simulink library "halout"  (R2021b)
settings: Solver=VariableStepAuto  StartTime=0.0  StopTime=10.0  RelTol=1e-3
undefined symbols (not defined in the file): C_TASK_5MS_S, FALSE, KHAL_CAN1TxReq_flg, KHAL_CAN2TxReq_flg, KHAL_CAN3FD3VCU1toNIDECTxReq_flg, KHAL_CAN3FD3VCU1TxReq_flg, KHAL_CAN3FD3VCU2E2E_flg, KHAL_CAN3FD3VCU2toNIDECE2E_flg, KHAL_CAN3FD3VCU2toNIDECTxReq_flg, KHAL_CAN3FD3VCU2TxReq_flg, KHAL_CAN3TxReq_flg, KHAL_CAN4FD4CE1000E2E_flg, KHAL_CAN4FD4CE1000TxReq_flg, KHAL_CAN4TxReq_flg, KHAL_CAN5TxReq_flg, KHAL_CAN7TxReq_flg, ONE_INT, TRUE, ZERO_INT
libraries: FVT_lib x258, simulink x115
(part 3 of 17)

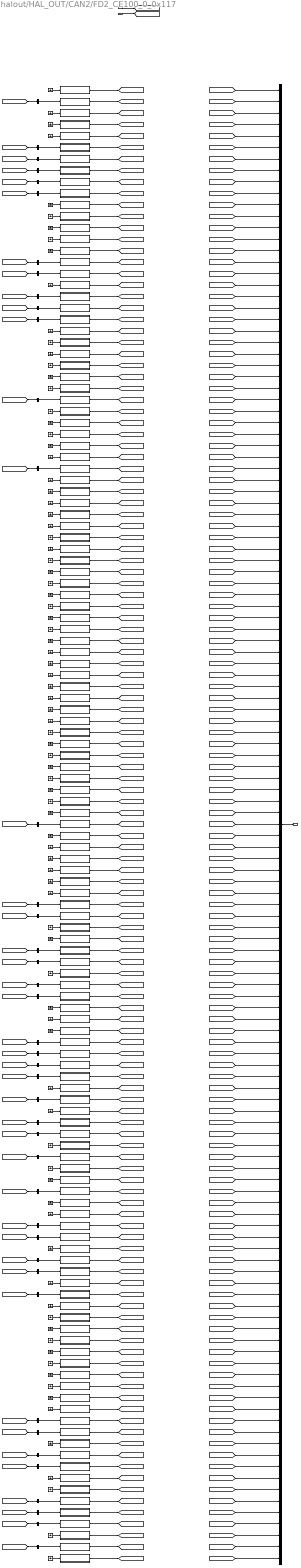
== system halout/HAL_OUT/CAN2/FD2_CE100_0_0x117 ==
  BSCP_outputs : Inport  OutDataTypeStr=Bus: BSCP_outputs
  BOUTP_outputs : Inport  Port=2  OutDataTypeStr=Bus: BOUTP_outputs
  APMDoorControlSta : Subsystem
  ActAPSPosn : Subsystem
  AllDoorSW : Subsystem
  AntitheftSta : Subsystem
  BCMDoorLockSta : Subsystem
  BrakeLamp : Subsystem
  CCCrlSta : Subsystem
  CCMSASpdWar : Subsystem
  CCUACLampSts : Subsystem
  CCUACMaxLampSts : Subsystem
  CCUAutoLampSts : Subsystem
  CCUAutoMidLampSts : Subsystem
  CCUDispalyRequest : Subsystem
  CCUEcoSts : Subsystem
  CCUFrtOnOffLampSts : Subsystem
  CCURrOnOffLampSts : Subsystem
  CCUSyncLampSts : Subsystem
  CoastDwModeStaChk : Subsystem
  CreepSWSta : Subsystem
  DISCButtSta : Subsystem
  DISCSta : Subsystem
  DemoModeStaChk : Subsystem
  Dimmer : Subsystem
  DimmerEN : Subsystem
  DisengagePFail : Subsystem
  DoorLockIND : Subsystem
  DrDoorSW : Subsystem
  DrSeatSta : Subsystem
  DynoModeStaChk : Subsystem
  EDriveSysErrAccPedalErr : Subsystem
  EDriveSysErrMCUErr : Subsystem
  EDriveSysErrShifterErr : Subsystem
  EDriveSysErrVCUErr : Subsystem
  EVDriveMode : Subsystem
  EngActvDmpDisabSta : Subsystem
  EngCoastDwSta : Subsystem
  EngPwrLockSta : Subsystem
  EngagePFail : Subsystem
  FDABSWarning : Subsystem
  FDBatteryChargeWarning : Subsystem
  FDCTHCMCLEVentYSta : Subsystem
  FDCTHCMCLEVentZSta : Subsystem
  FDCTHCMCLVentSta : Subsystem
  FDCTHCMCREVentYSta : Subsystem
  FDCTHCMCREVentZSta : Subsystem
  FDCTHCMCRVentSta : Subsystem
  FDCTHCMDrEVentModeSta : Subsystem
  FDCTHCMDrEVentYSta : Subsystem
  FDCTHCMDrEVentZSta : Subsystem
  FDCTHCMDrVentSta : Subsystem
  FDCTHCMPsEVentModeSta : Subsystem
  FDCTHCMPsEVentYSta : Subsystem
  FDCTHCMPsEVentZSta : Subsystem
  FDCTHCMPsVentSta : Subsystem
  FDCVCUPwrSaveReqCmd : Subsystem
  FDEDriveSystem : Subsystem
  FDEPBError : Subsystem
  FDHVBatteryFault : Subsystem
  FDParkBrakeWarning : Subsystem
  FDPowerlimitation : Subsystem
  FDSteeringWarning : Subsystem
  FDTCSIndicator : Subsystem
  FDTelltaleFail : Subsystem
  FalseNPreventSta : Subsystem
  FeatSetSpdFinalraw32 : Subsystem
  FollowMe : Subsystem
  FrFogLamp : Subsystem
  Ground{,1..86} (87 alike) : Ground
  HBeam : Subsystem
  HVRlyOpFail : Subsystem
  HVSysErrIsolationErr : Subsystem
  HVSysErrPackErr : Subsystem
  HVSysErrRelayErr : Subsystem
  HazardSW : Subsystem
  HoodSW : Subsystem
  LBSD : Subsystem
  LBeam : Subsystem
  LDRL : Subsystem
  LTurnLP : Subsystem
  LVChrgFuncStaChk : Subsystem
  LVSysErrPwrOutpErr : Subsystem
  LimphomeAct : Subsystem
  LockSetting : Subsystem
  MCUActDisFail : Subsystem
  MSACrlSta : Subsystem
  MeterIndSpeedraw32 : Subsystem
  PASStaFSys : Subsystem
  PosLamp : Subsystem
  PsDoorSW : Subsystem
  PwrSta : Subsystem
  PwrStaErr : Subsystem
  PwrStaONTOIVIPopReq : Subsystem
  PwrStaONTOIVIPopT : Subsystem
  RBSD : Subsystem
  RDRL : Subsystem
  RLDoorSW : Subsystem
  RRDoorSW : Subsystem
  RTurnLP : Subsystem
  ReqInternalV2LStatusLamp : Subsystem
  ReqV2LIVIPopup : Subsystem
  ReqV2LSwOn : Subsystem
  ReverseLamp : Subsystem
  RrDefog : Subsystem
  RrFogLamp : Subsystem
  ShiftGearPosn : Subsystem
  SysAllowReadySta : Subsystem
  SysPwrSta : Subsystem
  TailgateSW : Subsystem
  VCUBrkSWSta : Subsystem
  VCUFLDoorSta : Subsystem
  VCUFRDoorSta : Subsystem
  VCUHoodSWSta : Subsystem
  VCUOPDHold : Subsystem
  VCURLDoorSta : Subsystem
  VCURRDoorSta : Subsystem
  VCUTailgateSWSta : Subsystem
  VehMalfunLevel : Subsystem
  XWDMode : Subsystem
  bus_creator : BusCreator  Inputs=129  OutDataTypeStr=Bus: DT_CAN2_SG_FD2_CE100_0  NonVirtualBus=on
  bus_selector : BusSelector  OutputSignals=VOUTP_ActAPSPosn_pct
  bus_selector1 : BusSelector  OutputSignals=VOUTP_BrakeLamp_flg
  bus_selector10 : BusSelector  OutputSignals=VOUTP_DISCSta_enum
  bus_selector11 : BusSelector  OutputSignals=VOUTP_DrSeatSta_enum
  bus_selector12 : BusSelector  OutputSignals=VOUTP_EVDriveMode_enum
  bus_selector13 : BusSelector  OutputSignals=VOUTP_FeatSetSpdFinal_raw32
  bus_selector14 : BusSelector  OutputSignals=VOUTP_HBeam_flg
  bus_selector15 : BusSelector  OutputSignals=VOUTP_HazardSW_flg
  bus_selector16 : BusSelector  OutputSignals=VOUTP_LDRL_flg
  bus_selector17 : BusSelector  OutputSignals=VOUTP_LTurnLP_flg
  bus_selector18 : BusSelector  OutputSignals=VOUTP_LVSysErrPwrOutErr_flg
  bus_selector19 : BusSelector  OutputSignals=VOUTP_LBeam_flg
  bus_selector2 : BusSelector  OutputSignals=VOUTP_CCMSASpdWar_flg
  bus_selector20 : BusSelector  OutputSignals=VOUTP_MSACtrlSta_enum
  bus_selector21 : BusSelector  OutputSignals=VOUTP_MeterIndSpeed_raw32
  bus_selector22 : BusSelector  OutputSignals=VOUTP_StaFSya_flg
  bus_selector23 : BusSelector  OutputSignals=VOUTP_PosLamp_flg
  bus_selector24 : BusSelector  OutputSignals=VOUTP_PowerSta_enum
  bus_selector25 : BusSelector  OutputSignals=VOUTP_PwrStaONTOPopReq_flg
  bus_selector26 : BusSelector  OutputSignals=VOUTP_IVIPwrStaONTOPopT_s
  bus_selector27 : BusSelector  OutputSignals=VOUTP_RDRL_flg
  bus_selector28 : BusSelector  OutputSignals=VOUTP_RTurnLP_flg
  bus_selector29 : BusSelector  OutputSignals=VOUTP_ReqV2LIVIPopup_enum
  bus_selector3 : BusSelector  OutputSignals=VOUTP_CCUACLampSts_flg
  bus_selector30 : BusSelector  OutputSignals=VOUTP_ReverseLamp_flg
  bus_selector31 : BusSelector  OutputSignals=VOUTP_RrFogLamp_flg
  bus_selector32 : BusSelector  OutputSignals=VOUTP_ShiftGearPosn_enum
  bus_selector33 : BusSelector  OutputSignals=VOUTP_SysPowerMode_enum
  bus_selector34 : BusSelector  OutputSignals=VOUTP_DrivetrainSelect_enum
  bus_selector35 : BusSelector  OutputSignals=VOUTP_sigAirIntenZon1St_enum
  bus_selector36 : BusSelector  OutputSignals=VOUTP_sigAmbAirT_C
  bus_selector37 : BusSelector  OutputSignals=VOUTP_sigCbnAirT_C
  bus_selector38 : BusSelector  OutputSignals=VOUTP_sigRecircSt_flg
  bus_selector39 : BusSelector  OutputSignals=VOUTP_sigSetTempZon1St_C
  bus_selector4 : BusSelector  OutputSignals=VOUTP_CCUACMaxLampSts_flg
  bus_selector40 : BusSelector  OutputSignals=VOUTP_sigSetTempZon2St_C
  bus_selector41 : BusSelector  OutputSignals=VOUTP_sigWindDirZon1St_enum
  bus_selector5 : BusSelector  OutputSignals=VOUTP_CCUAutoLampSts_flg
  bus_selector6 : BusSelector  OutputSignals=VOUTP_CCUSyncLampSts_flg
  bus_selector7 : BusSelector  OutputSignals=VOUTP_CCCtrlSta_enum
  bus_selector8 : BusSelector  OutputSignals=VOUTP_CreepON_flg
  bus_selector9 : BusSelector  OutputSignals=VOUTP_DISCButtSta_flg
  sigAirIntenZon1St : Subsystem
  sigAirIntenZon3St : Subsystem
  sigAmbAirT : Subsystem
  sigCbnAirT : Subsystem
  sigDfrstSt : Subsystem
  sigHvacSt : Subsystem
  sigRecircSt : Subsystem
  sigSetTempZon1St : Subsystem
  sigSetTempZon2St : Subsystem
  sigSetTempZon3St : Subsystem
  sigWindDirZon1St : Subsystem
  sigWindDirZon3St : Subsystem
  FD2_CE100_0 : Outport
  wires:
  BSCP_outputs/1 -> [BSCP_outputs]
  BOUTP_outputs/1 -> [BOUTP_outputs]
  [CAN2_APMDoorControlSta] -> bus_creator/1  "CAN2_APMDoorControlSta"
  [CAN2_ActAPSPosn] -> bus_creator/2  "CAN2_ActAPSPosn"
  [CAN2_AllDoorSW] -> bus_creator/3  "CAN2_AllDoorSW"
  [CAN2_AntitheftSta] -> bus_creator/4  "CAN2_AntitheftSta"
  [CAN2_BCM_DoorLock_Sta] -> bus_creator/5  "CAN2_BCM_DoorLock_Sta"
  [CAN2_BrakeLamp] -> bus_creator/6  "CAN2_BrakeLamp"
  [CAN2_CCMSA_SpdWar] -> bus_creator/7  "CAN2_CCMSA_SpdWar"
  [CAN2_CCU_ACLampSts] -> bus_creator/8  "CAN2_CCU_ACLampSts"
  [CAN2_CCU_ACMaxLampSts] -> bus_creator/9  "CAN2_CCU_ACMaxLampSts"
  [CAN2_CCU_AutoLampSts] -> bus_creator/10  "CAN2_CCU_AutoLampSts"
  [CAN2_CCU_AutoMidLampSts] -> bus_creator/11  "CAN2_CCU_AutoMidLampSts"
  [CAN2_CCU_Dispaly_Request] -> bus_creator/12  "CAN2_CCU_Dispaly_Request"
  [CAN2_CCU_EcoSts] -> bus_creator/13  "CAN2_CCU_EcoSts"
  [CAN2_CCU_FrtOnOffLampSts] -> bus_creator/14  "CAN2_CCU_FrtOnOffLampSts"
  [CAN2_CCU_RrOnOffLampSts] -> bus_creator/15  "CAN2_CCU_RrOnOffLampSts"
  [CAN2_CCU_SyncLampSts] -> bus_creator/16  "CAN2_CCU_SyncLampSts"
  [CAN2_CC_Crl_Sta] -> bus_creator/17  "CAN2_CC_Crl_Sta"
  [CAN2_CoastDwModeStaChk] -> bus_creator/18  "CAN2_CoastDwModeStaChk"
  [CAN2_CreepSW_Sta] -> bus_creator/19  "CAN2_CreepSW_Sta"
  [CAN2_DISC_ButtSta] -> bus_creator/20  "CAN2_DISC_ButtSta"
  [CAN2_DISC_Sta] -> bus_creator/21  "CAN2_DISC_Sta"
  [CAN2_DemoModeStaChk] -> bus_creator/22  "CAN2_DemoModeStaChk"
  [CAN2_Dimmer] -> bus_creator/23  "CAN2_Dimmer"
  [CAN2_DimmerEN] -> bus_creator/24  "CAN2_DimmerEN"
  [CAN2_DisengageP_Fail] -> bus_creator/25  "CAN2_DisengageP_Fail"
  [CAN2_DoorLockIND] -> bus_creator/26  "CAN2_DoorLockIND"
  [CAN2_DrDoorSW] -> bus_creator/27  "CAN2_DrDoorSW"
  [CAN2_Dr_SeatSta] -> bus_creator/28  "CAN2_Dr_SeatSta"
  [CAN2_DynoModeStaChk] -> bus_creator/29  "CAN2_DynoModeStaChk"
  [CAN2_EDriveSysErr_AccPedalErr] -> bus_creator/30  "CAN2_EDriveSysErr_AccPedalErr"
  [CAN2_EDriveSysErr_MCUErr] -> bus_creator/31  "CAN2_EDriveSysErr_MCUErr"
  [CAN2_EDriveSysErr_ShifterErr] -> bus_creator/32  "CAN2_EDriveSysErr_ShifterErr"
  [CAN2_EDriveSysErr_VCUErr] -> bus_creator/33  "CAN2_EDriveSysErr_VCUErr"
  [CAN2_EVDriveMode] -> bus_creator/34  "CAN2_EVDriveMode"
  [CAN2_Eng_ActvDmpDisabSta] -> bus_creator/35  "CAN2_Eng_ActvDmpDisabSta"
  [CAN2_Eng_CoastDwSta] -> bus_creator/36  "CAN2_Eng_CoastDwSta"
  [CAN2_Eng_PwrLockSta] -> bus_creator/37  "CAN2_Eng_PwrLockSta"
  [CAN2_EngageP_Fail] -> bus_creator/38  "CAN2_EngageP_Fail"
  [CAN2_FDC_THCM_CLEVentY_Sta] -> bus_creator/39  "CAN2_FDC_THCM_CLEVentY_Sta"
  [CAN2_FDC_THCM_CLEVentZ_Sta] -> bus_creator/40  "CAN2_FDC_THCM_CLEVentZ_Sta"
  [CAN2_FDC_THCM_CLVent_Sta] -> bus_creator/41  "CAN2_FDC_THCM_CLVent_Sta"
  [CAN2_FDC_THCM_CREVentY_Sta] -> bus_creator/42  "CAN2_FDC_THCM_CREVentY_Sta"
  [CAN2_FDC_THCM_CREVentZ_Sta] -> bus_creator/43  "CAN2_FDC_THCM_CREVentZ_Sta"
  [CAN2_FDC_THCM_CRVent_Sta] -> bus_creator/44  "CAN2_FDC_THCM_CRVent_Sta"
  [CAN2_FDC_THCM_DrEVentMode_Sta] -> bus_creator/45  "CAN2_FDC_THCM_DrEVentMode_Sta"
  [CAN2_FDC_THCM_DrEVentY_Sta] -> bus_creator/46  "CAN2_FDC_THCM_DrEVentY_Sta"
  [CAN2_FDC_THCM_DrEVentZ_Sta] -> bus_creator/47  "CAN2_FDC_THCM_DrEVentZ_Sta"
  [CAN2_FDC_THCM_DrVent_Sta] -> bus_creator/48  "CAN2_FDC_THCM_DrVent_Sta"
  [CAN2_FDC_THCM_PsEVentMode_Sta] -> bus_creator/49  "CAN2_FDC_THCM_PsEVentMode_Sta"
  [CAN2_FDC_THCM_PsEVentY_Sta] -> bus_creator/50  "CAN2_FDC_THCM_PsEVentY_Sta"
  [CAN2_FDC_THCM_PsEVentZ_Sta] -> bus_creator/51  "CAN2_FDC_THCM_PsEVentZ_Sta"
  [CAN2_FDC_THCM_PsVent_Sta] -> bus_creator/52  "CAN2_FDC_THCM_PsVent_Sta"
  [CAN2_FDC_VCU_PwrSaveReq_Cmd] -> bus_creator/53  "CAN2_FDC_VCU_PwrSaveReq_Cmd"
  [CAN2_FD_ABS_Warning] -> bus_creator/54  "CAN2_FD_ABS_Warning"
  [CAN2_FD_Battery_Charge_Warning] -> bus_creator/55  "CAN2_FD_Battery_Charge_Warning"
  [CAN2_FD_EDrive_System] -> bus_creator/56  "CAN2_FD_EDrive_System"
  [CAN2_FD_EPB_Error] -> bus_creator/57  "CAN2_FD_EPB_Error"
  [CAN2_FD_HV_Battery_Fault] -> bus_creator/58  "CAN2_FD_HV_Battery_Fault"
  [CAN2_FD_Park_Brake_Warning] -> bus_creator/59  "CAN2_FD_Park_Brake_Warning"
  [CAN2_FD_Power_limitation] -> bus_creator/60  "CAN2_FD_Power_limitation"
  [CAN2_FD_Steering_Warning] -> bus_creator/61  "CAN2_FD_Steering_Warning"
  [CAN2_FD_TCS_Indicator] -> bus_creator/62  "CAN2_FD_TCS_Indicator"
  [CAN2_FD_Telltale_Fail] -> bus_creator/63  "CAN2_FD_Telltale_Fail"
  [CAN2_FalseNPrevent_Sta] -> bus_creator/64  "CAN2_FalseNPrevent_Sta"
  [CAN2_FeatSetSpdFinal_raw32] -> bus_creator/65  "CAN2_FeatSetSpdFinal_raw32"
  [CAN2_FollowMe] -> bus_creator/66  "CAN2_FollowMe"
  [CAN2_Fr_FogLamp] -> bus_creator/67  "CAN2_Fr_FogLamp"
  [CAN2_HVRlyOpFail] -> bus_creator/68  "CAN2_HVRlyOpFail"
  [CAN2_HVSysErr_IsolationErr] -> bus_creator/69  "CAN2_HVSysErr_IsolationErr"
  [CAN2_HVSysErr_PackErr] -> bus_creator/70  "CAN2_HVSysErr_PackErr"
  [CAN2_HVSysErr_RelayErr] -> bus_creator/71  "CAN2_HVSysErr_RelayErr"
  [CAN2_H_Beam] -> bus_creator/72  "CAN2_H_Beam"
  [CAN2_HazardSW] -> bus_creator/73  "CAN2_HazardSW"
  [CAN2_HoodSW] -> bus_creator/74  "CAN2_HoodSW"
  [CAN2_LBSD] -> bus_creator/75  "CAN2_LBSD"
  [CAN2_LDRL] -> bus_creator/76  "CAN2_LDRL"
  [CAN2_LTurnLP] -> bus_creator/77  "CAN2_LTurnLP"
  [CAN2_LVChrgFuncStaChk] -> bus_creator/78  "CAN2_LVChrgFuncStaChk"
  [CAN2_LVSysErr_PwrOutpErr] -> bus_creator/79  "CAN2_LVSysErr_PwrOutpErr"
  [CAN2_L_Beam] -> bus_creator/80  "CAN2_L_Beam"
  [CAN2_LimphomeAct] -> bus_creator/81  "CAN2_LimphomeAct"
  [CAN2_LockSetting] -> bus_creator/82  "CAN2_LockSetting"
  [CAN2_MCUActDisFail] -> bus_creator/83  "CAN2_MCUActDisFail"
  [CAN2_MSA_Crl_Sta] -> bus_creator/84  "CAN2_MSA_Crl_Sta"
  [CAN2_MeterIndSpeed_raw32] -> bus_creator/85  "CAN2_MeterIndSpeed_raw32"
  [CAN2_PAS_Sta_F_Sys] -> bus_creator/86  "CAN2_PAS_Sta_F_Sys"
  [CAN2_PosLamp] -> bus_creator/87  "CAN2_PosLamp"
  [CAN2_PsDoorSW] -> bus_creator/88  "CAN2_PsDoorSW"
  [CAN2_PwrSta] -> bus_creator/89  "CAN2_PwrSta"
  [CAN2_PwrStaErr] -> bus_creator/90  "CAN2_PwrStaErr"
  [CAN2_PwrStaONTOIVIPopReq] -> bus_creator/91  "CAN2_PwrStaONTOIVIPopReq"
  [CAN2_PwrStaONTOIVIPopT] -> bus_creator/92  "CAN2_PwrStaONTOIVIPopT"
  [CAN2_RBSD] -> bus_creator/93  "CAN2_RBSD"
  [CAN2_RDRL] -> bus_creator/94  "CAN2_RDRL"
  [CAN2_RLDoorSW] -> bus_creator/95  "CAN2_RLDoorSW"
  [CAN2_RRDoorSW] -> bus_creator/96  "CAN2_RRDoorSW"
  [CAN2_RTurnLP] -> bus_creator/97  "CAN2_RTurnLP"
  [CAN2_Req_Internal_V2L_Status_Lamp] -> bus_creator/98  "CAN2_Req_Internal_V2L_Status_Lamp"
  [CAN2_Req_V2LSwOn] -> bus_creator/99  "CAN2_Req_V2LSwOn"
  [CAN2_Req_V2L_IVI_Popup] -> bus_creator/100  "CAN2_Req_V2L_IVI_Popup"
  [CAN2_ReverseLamp] -> bus_creator/101  "CAN2_ReverseLamp"
  [CAN2_Rr_Defog] -> bus_creator/102  "CAN2_Rr_Defog"
  [CAN2_Rr_FogLamp] -> bus_creator/103  "CAN2_Rr_FogLamp"
  [CAN2_ShiftGearPosn] -> bus_creator/104  "CAN2_ShiftGearPosn"
  [CAN2_SysAllowReadySta] -> bus_creator/105  "CAN2_SysAllowReadySta"
  [CAN2_SysPwrSta] -> bus_creator/106  "CAN2_SysPwrSta"
  [CAN2_Tailgate_SW] -> bus_creator/107  "CAN2_Tailgate_SW"
  [CAN2_VCUBrkSWSta] -> bus_creator/108  "CAN2_VCUBrkSWSta"
  [CAN2_VCUFLDoorSta] -> bus_creator/109  "CAN2_VCUFLDoorSta"
  [CAN2_VCUFRDoorSta] -> bus_creator/110  "CAN2_VCUFRDoorSta"
  [CAN2_VCUHoodSWSta] -> bus_creator/111  "CAN2_VCUHoodSWSta"
  [CAN2_VCURLDoorSta] -> bus_creator/112  "CAN2_VCURLDoorSta"
  [CAN2_VCURRDoorSta] -> bus_creator/113  "CAN2_VCURRDoorSta"
  [CAN2_VCUTailgateSWSta] -> bus_creator/114  "CAN2_VCUTailgateSWSta"
  [CAN2_VCU_OPDHold] -> bus_creator/115  "CAN2_VCU_OPDHold"
  [CAN2_VehMalfunLevel] -> bus_creator/116  "CAN2_VehMalfunLevel"
  [CAN2_XWDMode] -> bus_creator/117  "CAN2_XWDMode"
  [CAN2_sigAirIntenZon1St] -> bus_creator/118  "CAN2_sigAirIntenZon1St"
  [CAN2_sigAirIntenZon3St] -> bus_creator/119  "CAN2_sigAirIntenZon3St"
  [CAN2_sigAmbAirT] -> bus_creator/120  "CAN2_sigAmbAirT"
  [CAN2_sigCbnAirT] -> bus_creator/121  "CAN2_sigCbnAirT"
  [CAN2_sigDfrstSt] -> bus_creator/122  "CAN2_sigDfrstSt"
  [CAN2_sigHvacSt] -> bus_creator/123  "CAN2_sigHvacSt"
  [CAN2_sigRecircSt] -> bus_creator/124  "CAN2_sigRecircSt"
  [CAN2_sigSetTempZon1St] -> bus_creator/125  "CAN2_sigSetTempZon1St"
  [CAN2_sigSetTempZon2St] -> bus_creator/126  "CAN2_sigSetTempZon2St"
  [CAN2_sigSetTempZon3St] -> bus_creator/127  "CAN2_sigSetTempZon3St"
  [CAN2_sigWindDirZon1St] -> bus_creator/128  "CAN2_sigWindDirZon1St"
  [CAN2_sigWindDirZon3St] -> bus_creator/129  "CAN2_sigWindDirZon3St"
  bus_creator/1 -> FD2_CE100_0/1
  APMDoorControlSta/1(CAN2_APMDoorControlSta) -> [CAN2_APMDoorControlSta]
  ActAPSPosn/1(CAN2_ActAPSPosn) -> [CAN2_ActAPSPosn]
  AllDoorSW/1(CAN2_AllDoorSW) -> [CAN2_AllDoorSW]
  AntitheftSta/1(CAN2_AntitheftSta) -> [CAN2_AntitheftSta]
  BCMDoorLockSta/1(CAN2_BCM_DoorLock_Sta) -> [CAN2_BCM_DoorLock_Sta]
  BrakeLamp/1(CAN2_BrakeLamp) -> [CAN2_BrakeLamp]
  CCMSASpdWar/1(CAN2_CCMSA_SpdWar) -> [CAN2_CCMSA_SpdWar]
  CCUACLampSts/1(CAN2_CCU_ACLampSts) -> [CAN2_CCU_ACLampSts]
  CCUACMaxLampSts/1(CAN2_CCU_ACMaxLampSts) -> [CAN2_CCU_ACMaxLampSts]
  CCUAutoLampSts/1(CAN2_CCU_AutoLampSts) -> [CAN2_CCU_AutoLampSts]
  CCUAutoMidLampSts/1(CAN2_CCU_AutoMidLampSts) -> [CAN2_CCU_AutoMidLampSts]
  CCUDispalyRequest/1(CAN2_CCU_Dispaly_Request) -> [CAN2_CCU_Dispaly_Request]
  CCUEcoSts/1(CAN2_CCU_EcoSts) -> [CAN2_CCU_EcoSts]
  CCUFrtOnOffLampSts/1(CAN2_CCU_FrtOnOffLampSts) -> [CAN2_CCU_FrtOnOffLampSts]
  CCURrOnOffLampSts/1(CAN2_CCU_RrOnOffLampSts) -> [CAN2_CCU_RrOnOffLampSts]
  CCUSyncLampSts/1(CAN2_CCU_SyncLampSts) -> [CAN2_CCU_SyncLampSts]
  CCCrlSta/1(CAN2_CC_Crl_Sta) -> [CAN2_CC_Crl_Sta]
  CoastDwModeStaChk/1(CAN2_CoastDwModeStaChk) -> [CAN2_CoastDwModeStaChk]
  CreepSWSta/1(CAN2_CreepSW_Sta) -> [CAN2_CreepSW_Sta]
  DISCButtSta/1(CAN2_DISC_ButtSta) -> [CAN2_DISC_ButtSta]
  DISCSta/1(CAN2_DISC_Sta) -> [CAN2_DISC_Sta]
  DemoModeStaChk/1(CAN2_DemoModeStaChk) -> [CAN2_DemoModeStaChk]
  Dimmer/1(CAN2_Dimmer) -> [CAN2_Dimmer]
  DimmerEN/1(CAN2_DimmerEN) -> [CAN2_DimmerEN]
  DisengagePFail/1(CAN2_DisengageP_Fail) -> [CAN2_DisengageP_Fail]
  DoorLockIND/1(CAN2_DoorLockIND) -> [CAN2_DoorLockIND]
  DrDoorSW/1(CAN2_DrDoorSW) -> [CAN2_DrDoorSW]
  DrSeatSta/1(CAN2_Dr_SeatSta) -> [CAN2_Dr_SeatSta]
  DynoModeStaChk/1(CAN2_DynoModeStaChk) -> [CAN2_DynoModeStaChk]
  EDriveSysErrAccPedalErr/1(CAN2_EDriveSysErr_AccPedalErr) -> [CAN2_EDriveSysErr_AccPedalErr]
  EDriveSysErrMCUErr/1(CAN2_EDriveSysErr_MCUErr) -> [CAN2_EDriveSysErr_MCUErr]
  EDriveSysErrShifterErr/1(CAN2_EDriveSysErr_ShifterErr) -> [CAN2_EDriveSysErr_ShifterErr]
  EDriveSysErrVCUErr/1(CAN2_EDriveSysErr_VCUErr) -> [CAN2_EDriveSysErr_VCUErr]
  EVDriveMode/1(CAN2_EVDriveMode) -> [CAN2_EVDriveMode]
  EngActvDmpDisabSta/1(CAN2_Eng_ActvDmpDisabSta) -> [CAN2_Eng_ActvDmpDisabSta]
  EngCoastDwSta/1(CAN2_Eng_CoastDwSta) -> [CAN2_Eng_CoastDwSta]
  EngPwrLockSta/1(CAN2_Eng_PwrLockSta) -> [CAN2_Eng_PwrLockSta]
  EngagePFail/1(CAN2_EngageP_Fail) -> [CAN2_EngageP_Fail]
  FDCTHCMCLEVentYSta/1(CAN2_FDC_THCM_CLEVentY_Sta) -> [CAN2_FDC_THCM_CLEVentY_Sta]
  FDCTHCMCLEVentZSta/1(CAN2_FDC_THCM_CLEVentZ_Sta) -> [CAN2_FDC_THCM_CLEVentZ_Sta]
  FDCTHCMCLVentSta/1(CAN2_FDC_THCM_CLVent_Sta) -> [CAN2_FDC_THCM_CLVent_Sta]
  FDCTHCMCREVentYSta/1(CAN2_FDC_THCM_CREVentY_Sta) -> [CAN2_FDC_THCM_CREVentY_Sta]
  FDCTHCMCREVentZSta/1(CAN2_FDC_THCM_CREVentZ_Sta) -> [CAN2_FDC_THCM_CREVentZ_Sta]
  FDCTHCMCRVentSta/1(CAN2_FDC_THCM_CRVent_Sta) -> [CAN2_FDC_THCM_CRVent_Sta]
  FDCTHCMDrEVentModeSta/1(CAN2_FDC_THCM_DrEVentMode_Sta) -> [CAN2_FDC_THCM_DrEVentMode_Sta]
  FDCTHCMDrEVentYSta/1(CAN2_FDC_THCM_DrEVentY_Sta) -> [CAN2_FDC_THCM_DrEVentY_Sta]
  FDCTHCMDrEVentZSta/1(CAN2_FDC_THCM_DrEVentZ_Sta) -> [CAN2_FDC_THCM_DrEVentZ_Sta]
  FDCTHCMDrVentSta/1(CAN2_FDC_THCM_DrVent_Sta) -> [CAN2_FDC_THCM_DrVent_Sta]
  FDCTHCMPsEVentModeSta/1(CAN2_FDC_THCM_PsEVentMode_Sta) -> [CAN2_FDC_THCM_PsEVentMode_Sta]
  FDCTHCMPsEVentYSta/1(CAN2_FDC_THCM_PsEVentY_Sta) -> [CAN2_FDC_THCM_PsEVentY_Sta]
  FDCTHCMPsEVentZSta/1(CAN2_FDC_THCM_PsEVentZ_Sta) -> [CAN2_FDC_THCM_PsEVentZ_Sta]
  FDCTHCMPsVentSta/1(CAN2_FDC_THCM_PsVent_Sta) -> [CAN2_FDC_THCM_PsVent_Sta]
  FDCVCUPwrSaveReqCmd/1(CAN2_FDC_VCU_PwrSaveReq_Cmd) -> [CAN2_FDC_VCU_PwrSaveReq_Cmd]
  FDABSWarning/1(CAN2_FD_ABS_Warning) -> [CAN2_FD_ABS_Warning]
  FDBatteryChargeWarning/1(CAN2_FD_Battery_Charge_Warning) -> [CAN2_FD_Battery_Charge_Warning]
  FDEDriveSystem/1(CAN2_FD_EDrive_System) -> [CAN2_FD_EDrive_System]
  FDEPBError/1(CAN2_FD_EPB_Error) -> [CAN2_FD_EPB_Error]
  FDHVBatteryFault/1(CAN2_FD_HV_Battery_Fault) -> [CAN2_FD_HV_Battery_Fault]
  FDParkBrakeWarning/1(CAN2_FD_Park_Brake_Warning) -> [CAN2_FD_Park_Brake_Warning]
  FDPowerlimitation/1(CAN2_FD_Power_limitation) -> [CAN2_FD_Power_limitation]
  FDSteeringWarning/1(CAN2_FD_Steering_Warning) -> [CAN2_FD_Steering_Warning]
  FDTCSIndicator/1(CAN2_FD_TCS_Indicator) -> [CAN2_FD_TCS_Indicator]
  FDTelltaleFail/1(CAN2_FD_Telltale_Fail) -> [CAN2_FD_Telltale_Fail]
  FalseNPreventSta/1(CAN2_FalseNPrevent_Sta) -> [CAN2_FalseNPrevent_Sta]
  FeatSetSpdFinalraw32/1(CAN2_FeatSetSpdFinal_raw32) -> [CAN2_FeatSetSpdFinal_raw32]
  FollowMe/1(CAN2_FollowMe) -> [CAN2_FollowMe]
  FrFogLamp/1(CAN2_Fr_FogLamp) -> [CAN2_Fr_FogLamp]
  HVRlyOpFail/1(CAN2_HVRlyOpFail) -> [CAN2_HVRlyOpFail]
  HVSysErrIsolationErr/1(CAN2_HVSysErr_IsolationErr) -> [CAN2_HVSysErr_IsolationErr]
  HVSysErrPackErr/1(CAN2_HVSysErr_PackErr) -> [CAN2_HVSysErr_PackErr]
  HVSysErrRelayErr/1(CAN2_HVSysErr_RelayErr) -> [CAN2_HVSysErr_RelayErr]
  HBeam/1(CAN2_H_Beam) -> [CAN2_H_Beam]
  HazardSW/1(CAN2_HazardSW) -> [CAN2_HazardSW]
  HoodSW/1(CAN2_HoodSW) -> [CAN2_HoodSW]
  LBSD/1(CAN2_LBSD) -> [CAN2_LBSD]
  LDRL/1(CAN2_LDRL) -> [CAN2_LDRL]
  LTurnLP/1(CAN2_LTurnLP) -> [CAN2_LTurnLP]
  LVChrgFuncStaChk/1(CAN2_LVChrgFuncStaChk) -> [CAN2_LVChrgFuncStaChk]
  LVSysErrPwrOutpErr/1(CAN2_LVSysErr_PwrOutpErr) -> [CAN2_LVSysErr_PwrOutpErr]
  LBeam/1(CAN2_L_Beam) -> [CAN2_L_Beam]
  LimphomeAct/1(CAN2_LimphomeAct) -> [CAN2_LimphomeAct]
  LockSetting/1(CAN2_LockSetting) -> [CAN2_LockSetting]
  MCUActDisFail/1(CAN2_MCUActDisFail) -> [CAN2_MCUActDisFail]
  MSACrlSta/1(CAN2_MSA_Crl_Sta) -> [CAN2_MSA_Crl_Sta]
  MeterIndSpeedraw32/1(CAN2_MeterIndSpeed_raw32) -> [CAN2_MeterIndSpeed_raw32]
  PASStaFSys/1(CAN2_PAS_Sta_F_Sys) -> [CAN2_PAS_Sta_F_Sys]
  PosLamp/1(CAN2_PosLamp) -> [CAN2_PosLamp]
  PsDoorSW/1(CAN2_PsDoorSW) -> [CAN2_PsDoorSW]
  PwrSta/1(CAN2_PwrSta) -> [CAN2_PwrSta]
  PwrStaErr/1(CAN2_PwrStaErr) -> [CAN2_PwrStaErr]
  PwrStaONTOIVIPopReq/1(CAN2_PwrStaONTOIVIPopReq) -> [CAN2_PwrStaONTOIVIPopReq]
  PwrStaONTOIVIPopT/1(CAN2_PwrStaONTOIVIPopT) -> [CAN2_PwrStaONTOIVIPopT]
  RBSD/1(CAN2_RBSD) -> [CAN2_RBSD]
  RDRL/1(CAN2_RDRL) -> [CAN2_RDRL]
  RLDoorSW/1(CAN2_RLDoorSW) -> [CAN2_RLDoorSW]
  RRDoorSW/1(CAN2_RRDoorSW) -> [CAN2_RRDoorSW]
  RTurnLP/1(CAN2_RTurnLP) -> [CAN2_RTurnLP]
  ReqInternalV2LStatusLamp/1(CAN2_Req_Internal_V2L_Status_Lamp) -> [CAN2_Req_Internal_V2L_Status_Lamp]
  ReqV2LSwOn/1(CAN2_Req_V2LSwOn) -> [CAN2_Req_V2LSwOn]
  ReqV2LIVIPopup/1(CAN2_Req_V2L_IVI_Popup) -> [CAN2_Req_V2L_IVI_Popup]
  ReverseLamp/1(CAN2_ReverseLamp) -> [CAN2_ReverseLamp]
  RrDefog/1(CAN2_Rr_Defog) -> [CAN2_Rr_Defog]
  RrFogLamp/1(CAN2_Rr_FogLamp) -> [CAN2_Rr_FogLamp]
  ShiftGearPosn/1(CAN2_ShiftGearPosn) -> [CAN2_ShiftGearPosn]
  SysAllowReadySta/1(CAN2_SysAllowReadySta) -> [CAN2_SysAllowReadySta]
  SysPwrSta/1(CAN2_SysPwrSta) -> [CAN2_SysPwrSta]
  TailgateSW/1(CAN2_Tailgate_SW) -> [CAN2_Tailgate_SW]
  VCUBrkSWSta/1(CAN2_VCUBrkSWSta) -> [CAN2_VCUBrkSWSta]
  VCUFLDoorSta/1(CAN2_VCUFLDoorSta) -> [CAN2_VCUFLDoorSta]
  VCUFRDoorSta/1(CAN2_VCUFRDoorSta) -> [CAN2_VCUFRDoorSta]
  VCUHoodSWSta/1(CAN2_VCUHoodSWSta) -> [CAN2_VCUHoodSWSta]
  VCURLDoorSta/1(CAN2_VCURLDoorSta) -> [CAN2_VCURLDoorSta]
  VCURRDoorSta/1(CAN2_VCURRDoorSta) -> [CAN2_VCURRDoorSta]
  VCUTailgateSWSta/1(CAN2_VCUTailgateSWSta) -> [CAN2_VCUTailgateSWSta]
  VCUOPDHold/1(CAN2_VCU_OPDHold) -> [CAN2_VCU_OPDHold]
  VehMalfunLevel/1(CAN2_VehMalfunLevel) -> [CAN2_VehMalfunLevel]
  XWDMode/1(CAN2_XWDMode) -> [CAN2_XWDMode]
  sigAirIntenZon1St/1(CAN2_sigAirIntenZon1St) -> [CAN2_sigAirIntenZon1St]
  sigAirIntenZon3St/1(CAN2_sigAirIntenZon3St) -> [CAN2_sigAirIntenZon3St]
  sigAmbAirT/1(CAN2_sigAmbAirT) -> [CAN2_sigAmbAirT]
  sigCbnAirT/1(CAN2_sigCbnAirT) -> [CAN2_sigCbnAirT]
  sigDfrstSt/1(CAN2_sigDfrstSt) -> [CAN2_sigDfrstSt]
  sigHvacSt/1(CAN2_sigHvacSt) -> [CAN2_sigHvacSt]
  sigRecircSt/1(CAN2_sigRecircSt) -> [CAN2_sigRecircSt]
  sigSetTempZon1St/1(CAN2_sigSetTempZon1St) -> [CAN2_sigSetTempZon1St]
  sigSetTempZon2St/1(CAN2_sigSetTempZon2St) -> [CAN2_sigSetTempZon2St]
  sigSetTempZon3St/1(CAN2_sigSetTempZon3St) -> [CAN2_sigSetTempZon3St]
  sigWindDirZon1St/1(CAN2_sigWindDirZon1St) -> [CAN2_sigWindDirZon1St]
  sigWindDirZon3St/1(CAN2_sigWindDirZon3St) -> [CAN2_sigWindDirZon3St]
  Ground/1 -> APMDoorControlSta/1(APMDoorControlSta)
  bus_selector/1 -> ActAPSPosn/1(ActAPSPosn)  "<VOUTP_ActAPSPosn_pct>"
  [BOUTP_outputs] -> bus_selector/1
  Ground1/1 -> AllDoorSW/1(AllDoorSW)
  Ground2/1 -> AntitheftSta/1(AntitheftSta)
  Ground3/1 -> BCMDoorLockSta/1(BCMDoorLockSta)
  bus_selector1/1 -> BrakeLamp/1(BrakeLamp)  "<VOUTP_BrakeLamp_flg>"
  [BOUTP_outputs] -> bus_selector1/1
  bus_selector2/1 -> CCMSASpdWar/1(CCMSASpdWar)  "<VOUTP_CCMSASpdWar_flg>"
  [BOUTP_outputs] -> bus_selector2/1
  bus_selector3/1 -> CCUACLampSts/1(CCUACLampSts)  "<VOUTP_CCUACLampSts_flg>"
  [BOUTP_outputs] -> bus_selector3/1
  bus_selector4/1 -> CCUACMaxLampSts/1(CCUACMaxLampSts)  "<VOUTP_CCUACMaxLampSts_flg>"
  [BOUTP_outputs] -> bus_selector4/1
  bus_selector5/1 -> CCUAutoLampSts/1(CCUAutoLampSts)  "<VOUTP_CCUAutoLampSts_flg>"
  [BOUTP_outputs] -> bus_selector5/1
  Ground4/1 -> CCUAutoMidLampSts/1(CCUAutoMidLampSts)
  Ground5/1 -> CCUDispalyRequest/1(CCUDispalyRequest)
  Ground6/1 -> CCUEcoSts/1(CCUEcoSts)
  Ground7/1 -> CCUFrtOnOffLampSts/1(CCUFrtOnOffLampSts)
  Ground8/1 -> CCURrOnOffLampSts/1(CCURrOnOffLampSts)
  bus_selector6/1 -> CCUSyncLampSts/1(CCUSyncLampSts)  "<VOUTP_CCUSyncLampSts_flg>"
  [BOUTP_outputs] -> bus_selector6/1
  bus_selector7/1 -> CCCrlSta/1(CCCrlSta)  "<VOUTP_CCCtrlSta_enum>"
  [BOUTP_outputs] -> bus_selector7/1
  Ground9/1 -> CoastDwModeStaChk/1(CoastDwModeStaChk)
  bus_selector8/1 -> CreepSWSta/1(CreepSWSta)  "<VOUTP_CreepON_flg>"
  [BOUTP_outputs] -> bus_selector8/1
  bus_selector9/1 -> DISCButtSta/1(DISCButtSta)  "<VOUTP_DISCButtSta_flg>"
  [BOUTP_outputs] -> bus_selector9/1
  bus_selector10/1 -> DISCSta/1(DISCSta)  "<VOUTP_DISCSta_enum>"
  [BOUTP_outputs] -> bus_selector10/1
  Ground10/1 -> DemoModeStaChk/1(DemoModeStaChk)
  Ground11/1 -> Dimmer/1(Dimmer)
  Ground12/1 -> DimmerEN/1(DimmerEN)
  Ground13/1 -> DisengagePFail/1(DisengagePFail)
  Ground14/1 -> DoorLockIND/1(DoorLockIND)
  Ground15/1 -> DrDoorSW/1(DrDoorSW)
  bus_selector11/1 -> DrSeatSta/1(DrSeatSta)  "<VOUTP_DrSeatSta_enum>"
  [BOUTP_outputs] -> bus_selector11/1
  Ground16/1 -> DynoModeStaChk/1(DynoModeStaChk)
  Ground17/1 -> EDriveSysErrAccPedalErr/1(EDriveSysErrAccPedalErr)
  Ground18/1 -> EDriveSysErrMCUErr/1(EDriveSysErrMCUErr)
  Ground19/1 -> EDriveSysErrShifterErr/1(EDriveSysErrShifterErr)
  Ground20/1 -> EDriveSysErrVCUErr/1(EDriveSysErrVCUErr)
  bus_selector12/1 -> EVDriveMode/1(EVDriveMode)  "<VOUTP_EVDriveMode_enum>"
  [BOUTP_outputs] -> bus_selector12/1
  Ground21/1 -> EngActvDmpDisabSta/1(EngActvDmpDisabSta)
  Ground22/1 -> EngCoastDwSta/1(EngCoastDwSta)
  Ground23/1 -> EngPwrLockSta/1(EngPwrLockSta)
  Ground24/1 -> EngagePFail/1(EngagePFail)
  Ground25/1 -> FDCTHCMCLEVentYSta/1(FDCTHCMCLEVentYSta)
  Ground26/1 -> FDCTHCMCLEVentZSta/1(FDCTHCMCLEVentZSta)
  Ground27/1 -> FDCTHCMCLVentSta/1(FDCTHCMCLVentSta)
  Ground28/1 -> FDCTHCMCREVentYSta/1(FDCTHCMCREVentYSta)
  Ground29/1 -> FDCTHCMCREVentZSta/1(FDCTHCMCREVentZSta)
  Ground30/1 -> FDCTHCMCRVentSta/1(FDCTHCMCRVentSta)
  Ground31/1 -> FDCTHCMDrEVentModeSta/1(FDCTHCMDrEVentModeSta)
  Ground32/1 -> FDCTHCMDrEVentYSta/1(FDCTHCMDrEVentYSta)
  Ground33/1 -> FDCTHCMDrEVentZSta/1(FDCTHCMDrEVentZSta)
  Ground34/1 -> FDCTHCMDrVentSta/1(FDCTHCMDrVentSta)
  Ground35/1 -> FDCTHCMPsEVentModeSta/1(FDCTHCMPsEVentModeSta)
  Ground36/1 -> FDCTHCMPsEVentYSta/1(FDCTHCMPsEVentYSta)
  Ground37/1 -> FDCTHCMPsEVentZSta/1(FDCTHCMPsEVentZSta)
  Ground38/1 -> FDCTHCMPsVentSta/1(FDCTHCMPsVentSta)
  Ground39/1 -> FDCVCUPwrSaveReqCmd/1(FDCVCUPwrSaveReqCmd)
  Ground40/1 -> FDABSWarning/1(FDABSWarning)
  Ground41/1 -> FDBatteryChargeWarning/1(FDBatteryChargeWarning)
  Ground42/1 -> FDEDriveSystem/1(FDEDriveSystem)
  Ground43/1 -> FDEPBError/1(FDEPBError)
  Ground44/1 -> FDHVBatteryFault/1(FDHVBatteryFault)
  Ground45/1 -> FDParkBrakeWarning/1(FDParkBrakeWarning)
  Ground46/1 -> FDPowerlimitation/1(FDPowerlimitation)
  Ground47/1 -> FDSteeringWarning/1(FDSteeringWarning)
  Ground48/1 -> FDTCSIndicator/1(FDTCSIndicator)
  Ground49/1 -> FDTelltaleFail/1(FDTelltaleFail)
  Ground50/1 -> FalseNPreventSta/1(FalseNPreventSta)
  bus_selector13/1 -> FeatSetSpdFinalraw32/1(FeatSetSpdFinalraw32)  "<VOUTP_FeatSetSpdFinal_raw32>"
  [BOUTP_outputs] -> bus_selector13/1
  Ground51/1 -> FollowMe/1(FollowMe)
  Ground52/1 -> FrFogLamp/1(FrFogLamp)
  Ground53/1 -> HVRlyOpFail/1(HVRlyOpFail)
  Ground54/1 -> HVSysErrIsolationErr/1(HVSysErrIsolationErr)
  Ground55/1 -> HVSysErrPackErr/1(HVSysErrPackErr)
  Ground56/1 -> HVSysErrRelayErr/1(HVSysErrRelayErr)
  bus_selector14/1 -> HBeam/1(HBeam)  "<VOUTP_HBeam_flg>"
  [BOUTP_outputs] -> bus_selector14/1
  bus_selector15/1 -> HazardSW/1(HazardSW)  "<VOUTP_HazardSW_flg>"
  [BOUTP_outputs] -> bus_selector15/1
  Ground57/1 -> HoodSW/1(HoodSW)
  Ground58/1 -> LBSD/1(LBSD)
  bus_selector16/1 -> LDRL/1(LDRL)  "<VOUTP_LDRL_flg>"
  [BOUTP_outputs] -> bus_selector16/1
  bus_selector17/1 -> LTurnLP/1(LTurnLP)  "<VOUTP_LTurnLP_flg>"
  [BOUTP_outputs] -> bus_selector17/1
  Ground59/1 -> LVChrgFuncStaChk/1(LVChrgFuncStaChk)
  bus_selector18/1 -> LVSysErrPwrOutpErr/1(LVSysErrPwrOutpErr)  "<VOUTP_LVSysErrPwrOutErr_flg>"
  [BOUTP_outputs] -> bus_selector18/1
  bus_selector19/1 -> LBeam/1(LBeam)  "<VOUTP_LBeam_flg>"
  [BOUTP_outputs] -> bus_selector19/1
  Ground60/1 -> LimphomeAct/1(LimphomeAct)
  Ground61/1 -> LockSetting/1(LockSetting)
  Ground62/1 -> MCUActDisFail/1(MCUActDisFail)
  bus_selector20/1 -> MSACrlSta/1(MSACrlSta)  "<VOUTP_MSACtrlSta_enum>"
  [BOUTP_outputs] -> bus_selector20/1
  bus_selector21/1 -> MeterIndSpeedraw32/1(MeterIndSpeedraw32)  "<VOUTP_MeterIndSpeed_raw32>"
  [BOUTP_outputs] -> bus_selector21/1
  bus_selector22/1 -> PASStaFSys/1(PASStaFSys)  "<VOUTP_StaFSya_flg>"
  [BOUTP_outputs] -> bus_selector22/1
  bus_selector23/1 -> PosLamp/1(PosLamp)  "<VOUTP_PosLamp_flg>"
  [BOUTP_outputs] -> bus_selector23/1
  Ground63/1 -> PsDoorSW/1(PsDoorSW)
  bus_selector24/1 -> PwrSta/1(PwrSta)  "<VOUTP_PowerSta_enum>"
  [BOUTP_outputs] -> bus_selector24/1
  Ground64/1 -> PwrStaErr/1(PwrStaErr)
  bus_selector25/1 -> PwrStaONTOIVIPopReq/1(PwrStaONTOIVIPopReq)  "<VOUTP_PwrStaONTOPopReq_flg>"
  [BOUTP_outputs] -> bus_selector25/1
  bus_selector26/1 -> PwrStaONTOIVIPopT/1(PwrStaONTOIVIPopT)  "<VOUTP_IVIPwrStaONTOPopT_s>"
  [BOUTP_outputs] -> bus_selector26/1
  Ground65/1 -> RBSD/1(RBSD)
  bus_selector27/1 -> RDRL/1(RDRL)  "<VOUTP_RDRL_flg>"
  [BOUTP_outputs] -> bus_selector27/1
  Ground66/1 -> RLDoorSW/1(RLDoorSW)
  Ground67/1 -> RRDoorSW/1(RRDoorSW)
  bus_selector28/1 -> RTurnLP/1(RTurnLP)  "<VOUTP_RTurnLP_flg>"
  [BOUTP_outputs] -> bus_selector28/1
  Ground68/1 -> ReqInternalV2LStatusLamp/1(ReqInternalV2LStatusLamp)
  Ground69/1 -> ReqV2LSwOn/1(ReqV2LSwOn)
  bus_selector29/1 -> ReqV2LIVIPopup/1(ReqV2LIVIPopup)  "<VOUTP_ReqV2LIVIPopup_enum>"
  [BOUTP_outputs] -> bus_selector29/1
  bus_selector30/1 -> ReverseLamp/1(ReverseLamp)  "<VOUTP_ReverseLamp_flg>"
  [BOUTP_outputs] -> bus_selector30/1
  Ground70/1 -> RrDefog/1(RrDefog)
  bus_selector31/1 -> RrFogLamp/1(RrFogLamp)  "<VOUTP_RrFogLamp_flg>"
  [BOUTP_outputs] -> bus_selector31/1
  bus_selector32/1 -> ShiftGearPosn/1(ShiftGearPosn)  "<VOUTP_ShiftGearPosn_enum>"
  [BOUTP_outputs] -> bus_selector32/1
  Ground71/1 -> SysAllowReadySta/1(SysAllowReadySta)
  bus_selector33/1 -> SysPwrSta/1(SysPwrSta)  "<VOUTP_SysPowerMode_enum>"
  [BOUTP_outputs] -> bus_selector33/1
  Ground72/1 -> TailgateSW/1(TailgateSW)
  Ground73/1 -> VCUBrkSWSta/1(VCUBrkSWSta)
  Ground74/1 -> VCUFLDoorSta/1(VCUFLDoorSta)
  Ground75/1 -> VCUFRDoorSta/1(VCUFRDoorSta)
  Ground76/1 -> VCUHoodSWSta/1(VCUHoodSWSta)
  Ground77/1 -> VCURLDoorSta/1(VCURLDoorSta)
  Ground78/1 -> VCURRDoorSta/1(VCURRDoorSta)
  Ground79/1 -> VCUTailgateSWSta/1(VCUTailgateSWSta)
  Ground80/1 -> VCUOPDHold/1(VCUOPDHold)
  Ground81/1 -> VehMalfunLevel/1(VehMalfunLevel)
  bus_selector34/1 -> XWDMode/1(XWDMode)  "<VOUTP_DrivetrainSelect_enum>"
  [BOUTP_outputs] -> bus_selector34/1
  bus_selector35/1 -> sigAirIntenZon1St/1(sigAirIntenZon1St)  "<VOUTP_sigAirIntenZon1St_enum>"
  [BOUTP_outputs] -> bus_selector35/1
  Ground82/1 -> sigAirIntenZon3St/1(sigAirIntenZon3St)
  bus_selector36/1 -> sigAmbAirT/1(sigAmbAirT)  "<VOUTP_sigAmbAirT_C>"
  [BOUTP_outputs] -> bus_selector36/1
  bus_selector37/1 -> sigCbnAirT/1(sigCbnAirT)  "<VOUTP_sigCbnAirT_C>"
  [BOUTP_outputs] -> bus_selector37/1
  Ground83/1 -> sigDfrstSt/1(sigDfrstSt)
  Ground84/1 -> sigHvacSt/1(sigHvacSt)
  bus_selector38/1 -> sigRecircSt/1(sigRecircSt)  "<VOUTP_sigRecircSt_flg>"
  [BOUTP_outputs] -> bus_selector38/1
  bus_selector39/1 -> sigSetTempZon1St/1(sigSetTempZon1St)  "<VOUTP_sigSetTempZon1St_C>"
  [BOUTP_outputs] -> bus_selector39/1
  bus_selector40/1 -> sigSetTempZon2St/1(sigSetTempZon2St)  "<VOUTP_sigSetTempZon2St_C>"
  [BOUTP_outputs] -> bus_selector40/1
  Ground85/1 -> sigSetTempZon3St/1(sigSetTempZon3St)
  bus_selector41/1 -> sigWindDirZon1St/1(sigWindDirZon1St)  "<VOUTP_sigWindDirZon1St_enum>"
  [BOUTP_outputs] -> bus_selector41/1
  Ground86/1 -> sigWindDirZon3St/1(sigWindDirZon3St)

== system halout/HAL_OUT/CAN2/FD2_CE100_1_0x202 ==
  BSCP_outputs : Inport  OutDataTypeStr=Bus: BSCP_outputs
  BOUTP_outputs : Inport  Port=2  OutDataTypeStr=Bus: BOUTP_outputs
  FDCBCMTgateSWLSta : Subsystem
  FDCBCMTgateSWRSta : Subsystem
  FDCBCMWelcomeDemoSta : Subsystem
  FDCVCUDACStatusSta : Subsystem
  FDCVCUTUpAStaSta : Subsystem
  bus_creator : BusCreator  Inputs=5  OutDataTypeStr=Bus: DT_CAN2_SG_FD2_CE100_1  NonVirtualBus=on
  bus_selector : BusSelector  OutputSignals=VOUTP_TgateSWLSta_flg
  bus_selector1 : BusSelector  OutputSignals=VOUTP_TgateSWRSta_flg
  bus_selector2 : BusSelector  OutputSignals=VOUTP_WelcomeDemoSta_flg
  bus_selector3 : BusSelector  OutputSignals=VOUTP_FDCVCUDACStatusSta_enum
  bus_selector4 : BusSelector  OutputSignals=VOUTP_FDCVCUTUpAStaSta_enum
  FD2_CE100_1 : Outport
  wires:
  BSCP_outputs/1 -> [BSCP_outputs]
  BOUTP_outputs/1 -> [BOUTP_outputs]
  [CAN2_FDC_BCM_TgateSWL_Sta] -> bus_creator/1  "CAN2_FDC_BCM_TgateSWL_Sta"
  [CAN2_FDC_BCM_TgateSWR_Sta] -> bus_creator/2  "CAN2_FDC_BCM_TgateSWR_Sta"
  [CAN2_FDC_BCM_WelcomeDemo_Sta] -> bus_creator/3  "CAN2_FDC_BCM_WelcomeDemo_Sta"
  [CAN2_FDC_VCU_DACStatus_Sta] -> bus_creator/4  "CAN2_FDC_VCU_DACStatus_Sta"
  [CAN2_FDC_VCU_TUpASta_Sta] -> bus_creator/5  "CAN2_FDC_VCU_TUpASta_Sta"
  bus_creator/1 -> FD2_CE100_1/1
  FDCBCMTgateSWLSta/1(CAN2_FDC_BCM_TgateSWL_Sta) -> [CAN2_FDC_BCM_TgateSWL_Sta]
  FDCBCMTgateSWRSta/1(CAN2_FDC_BCM_TgateSWR_Sta) -> [CAN2_FDC_BCM_TgateSWR_Sta]
  FDCBCMWelcomeDemoSta/1(CAN2_FDC_BCM_WelcomeDemo_Sta) -> [CAN2_FDC_BCM_WelcomeDemo_Sta]
  FDCVCUDACStatusSta/1(CAN2_FDC_VCU_DACStatus_Sta) -> [CAN2_FDC_VCU_DACStatus_Sta]
  FDCVCUTUpAStaSta/1(CAN2_FDC_VCU_TUpASta_Sta) -> [CAN2_FDC_VCU_TUpASta_Sta]
  bus_selector/1 -> FDCBCMTgateSWLSta/1(FDCBCMTgateSWLSta)  "<VOUTP_TgateSWLSta_flg>"
  [BOUTP_outputs] -> bus_selector/1
  bus_selector1/1 -> FDCBCMTgateSWRSta/1(FDCBCMTgateSWRSta)  "<VOUTP_TgateSWRSta_flg>"
  [BOUTP_outputs] -> bus_selector1/1
  bus_selector2/1 -> FDCBCMWelcomeDemoSta/1(FDCBCMWelcomeDemoSta)  "<VOUTP_WelcomeDemoSta_flg>"
  [BOUTP_outputs] -> bus_selector2/1
  bus_selector3/1 -> FDCVCUDACStatusSta/1(FDCVCUDACStatusSta)  "<VOUTP_FDCVCUDACStatusSta_enum>"
  [BOUTP_outputs] -> bus_selector3/1
  bus_selector4/1 -> FDCVCUTUpAStaSta/1(FDCVCUTUpAStaSta)  "<VOUTP_FDCVCUTUpAStaSta_enum>"
  [BOUTP_outputs] -> bus_selector4/1
